simulink model "Final_test"  (R2018a)
settings: Solver=FixedStepAuto  StartTime=0.0  StopTime=inf  FixedStep=0.01  RelTol=1e-3  EnableMultiTasking=on
InitFcn:
  | set_param('Final_test/Output/Run Sim','Value','1');
  | set_param('Final_test/Motor Switch','Value','0');
  | set_param('Final_test/Automatic Control','Value','0');
  | %set_param('Final_test/Manual PWM','Gain','0');
undefined symbols (not defined in the file or in its folder): Discrete, sigbuilder_block, Time
libraries: simulink x3, arduinolib x3, ctrlSharedLib x1, dspstat3 x1
settings Model: SimulationMode=external  ExtModeTrigDuration=2  Creator=adiravishankara  LastModifiedBy=adiravishankara
settings SolverCC: AutoInsertRateTranBlk=on
settings OptimizationCC: EnhancedBackFolding=on  PassReuseOutputArgsThreshold=0  MaxStackSize=64  OptimizeBlockOrder=speed  DifferentSizesBufferReuse=on  OptimizationCustomize=off
settings DebuggingCC: ParameterTunabilityLossMsg=error
settings HardwareCC: ProdBitPerPointer=32  ProdBitPerSizeT=32  ProdBitPerPtrDiffT=32  ProdLargestAtomicInteger=Long  ProdLargestAtomicFloat=Double  ProdWordSize=32  ProdHWDeviceType=ARM Compatible->ARM Cortex  UseEmbeddedCoderFeatures=off
settings SFSimCC: MATLABDynamicMemAlloc=off
settings RTWCC: SystemTargetFile=ert.tlc  HardwareBoard=Arduino Due  TLCOptions=-aInlineSetEventsForThisBaseRateFcn=TLC_FALSE -aSuppressMultiTaskScheduler=TLC_FALSE -aRateBasedStepFcn=1  TemplateMakefile=ert_default_tmf  GenerateReport=on  Toolchain=Arduino ARM  BuildConfiguration=Faster Runs  LaunchReport=on
settings CodeAppCC: ForceParamTrailComments=on  OperatorAnnotations=on
settings ERTTargetCC: ERTCustomFileBanners=off  SupportContinuousTime=on  SupportNonInlinedSFcns=on  RemoveResetFunc=off  SupportVariableSizeSignals=on  ModelStepFunctionPrototypeControlCompliant=off  ExtMode=on  ExtModeMexArgs='127.0.0.1' 0 17725  ERTSrcFileBannerTemplate=codertarget_code_template.cgt  ERTHdrFileBannerTemplate=codertarget_code_template.cgt  ERTDataSrcFileTemplate=codertarget_code_template.cgt  ERTDataHdrFileTemplate=codertarget_code_template.cgt

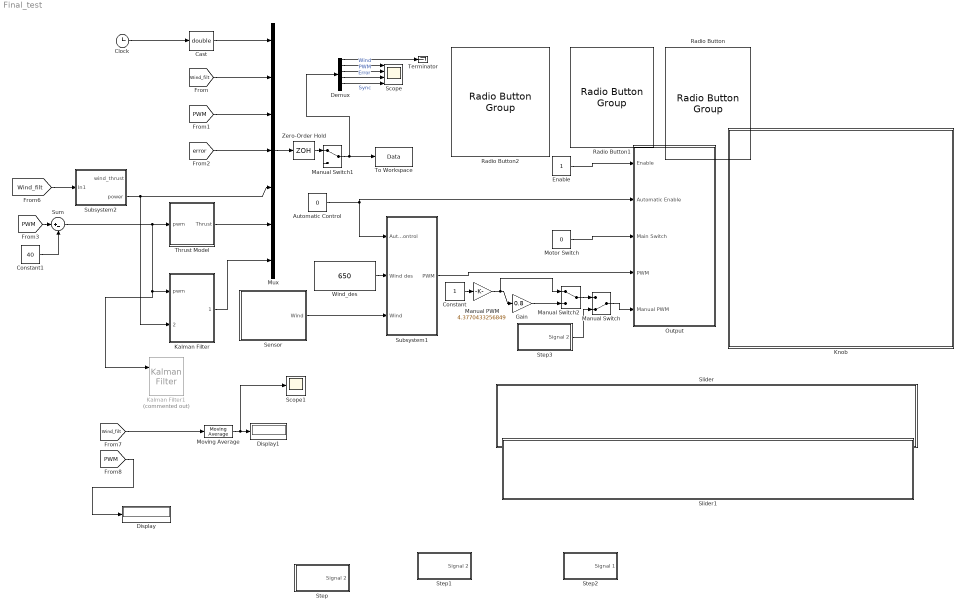
== system Final_test ==
  Automatic Control : Constant  Value=0  SampleTime=0.01
  Cast : DataTypeConversion  OutDataTypeStr=double
  Clock : Clock
  Constant : Constant  SampleTime=0.01
  Constant1 : Constant  Value=40
  Demux : Demux  Outputs=6
  Display : Display
  Display1 : Display
  Enable : Constant  SampleTime=0.01
  Gain : Gain  Gain=0.8
  Kalman Filter : Subsystem
  Kalman Filter1 : ctrlSharedLib/Kalman Filter  Commented=on  TimeDomain=Discrete-Time  UseCurrentEstimator=on  ModelSource=Individual A, B, C, D matrices  ModelSourceVariable=ss(0.95,1,1,0,1)  A="[0.9998  0.009851; -0.0394    0.9702]"  B=[0.000198; 0.0394]  C=[1 0]  D=0  NumberOfStates=1  NumberOfInputs=1  NumberOfOutputs=1  InitialEstimateSource=Dialog  X0=0  P0=10  UseK=off  UseGH=off  NumberOfProcessNoiseInputs=1  G=1  TimeInvariantG=on  H=0  TimeInvariantH=on  Q=1  TimeInvariantQ=on  R=5  TimeInvariantR=on  N=0  TimeInvariantN=on  AddInputPort=on  AddEnablePort=off  OutputEstimatedY=off  OutputP=off  Ts=-1
      settings: SourceProductBaseCode=CT
  Knob : Subsystem  DialogController=hmiCreateDDGDialog  IsWebBlock=on  mask(MWDashboardBlock){webBlockId=852d3d9e-f600-4180-8955-96c4171a0510, webBlockType=continuousknob, ShowInLibBrowser=on, ShowInitialText=on, HMISrcModelName=Final_test}
      mask prompts: webBlockId "WebBlock Id"; webBlockType "WebBlock Type"; HMISrcModelName "Source Model"
      mask help: SimulinkHMI:dialogs:ContinuousKnobDialogDesc
      mask Help: helpview([docroot '/mapfiles/simulink.map'], 'hmi_knob')
      mask Display:
      | if strcmp(get_param(bdroot(gcb),'BlockDiagramType'), 'library')
      |     image([(matlabroot) '/toolbox/simulink/hmi/icons/ContinuousKnob.png']);
      | end
  Manual PWM : Gain  Gain=4.3770433256849
  Manual Switch : ManualSwitch  CurrentSetting=0
  Manual Switch1 : ManualSwitch
  Manual Switch2 : ManualSwitch
  Motor Switch : Constant  Value=0  SampleTime=0.01
  Moving Average : dspstat3/Moving Average  Method=Sliding window  ForgettingFactorPort=off  SpecifyWindowLength=on  WindowLength=5  ForgettingFactor=0.9  SimulateUsing=Code generation
  Mux : Mux  Inputs=7
  Output : Subsystem
  Radio Button : RadioButtonGroup  WebBlockId=124  SelectedLabel=OFF  ButtonGroupName=SIM STATUS
      settings: Values={{'ON', 'OFF'}, [1 0]}
  Radio Button1 : RadioButtonGroup  WebBlockId=141  SelectedLabel=OFF  ButtonGroupName=SIM STATUS
      settings: Values={{'ON', 'OFF'}, [1 0]}
  Radio Button2 : RadioButtonGroup  WebBlockId=144  SelectedLabel=OFF  ButtonGroupName=SIM STATUS
      settings: Values={{'ON', 'OFF'}, [1 0]}
  Scope : Scope  NumInputPorts=4
  Scope1 : Scope
  Sensor : Subsystem
  Slider : Subsystem  DialogController=hmiCreateDDGDialog  IsWebBlock=on  mask(MWDashboardBlock){webBlockId=6d6bce73-9061-4720-a103-f9820fa904f8, webBlockType=slider, ShowInLibBrowser=on, ShowInitialText=on, HMISrcModelName=Final_test}
      mask prompts: webBlockId "WebBlock Id"; webBlockType "WebBlock Type"; HMISrcModelName "Source Model"
      mask help: SimulinkHMI:dialogs:SliderDialogDesc
      mask Help: helpview([docroot '/mapfiles/simulink.map'], 'hmi_slider')
      mask Display:
      | if strcmp(get_param(bdroot(gcb),'BlockDiagramType'), 'library')
      |     image([(matlabroot) '/toolbox/simulink/hmi/icons/Slider.png']);
      | end
  Slider1 : Subsystem  DialogController=hmiCreateDDGDialog  IsWebBlock=on  mask(MWDashboardBlock){webBlockId=583235cf-a666-476d-a93b-c374fcd1b609, webBlockType=slider, ShowInLibBrowser=on, ShowInitialText=on, HMISrcModelName=Final_test}
      mask prompts: webBlockId "WebBlock Id"; webBlockType "WebBlock Type"; HMISrcModelName "Source Model"
      mask help: SimulinkHMI:dialogs:SliderDialogDesc
      mask Help: helpview([docroot '/mapfiles/simulink.map'], 'hmi_slider')
      mask Display:
      | if strcmp(get_param(bdroot(gcb),'BlockDiagramType'), 'library')
      |     image([(matlabroot) '/toolbox/simulink/hmi/icons/Slider.png']);
      | end
  Step : Subsystem  Tag=STV Subsys  LoadFcn=sigbuilder_block('load');  StartFcn=sigbuilder_block('start');  StopFcn=sigbuilder_block('stop');  ClipboardFcn=sigbuilder_block('clipboard');  mask(Sigbuilder block){tuvar=[0:10]}
      mask help: Simulink:masks:SigbuilderBlock_MD
      mask init:
      | if ~strcmp(get_param(bdroot(gcbh),'SimulationStatus'),'stopped') tuvar = sigbuilder_block('maskInit'); end
      settings: CopyFcn=sigbuilder_block('copy');  DeleteFcn=sigbuilder_block('delete');  ModelCloseFcn=sigbuilder_block('modelClose');  PreSaveFcn=sigbuilder_block('preSave');  PauseFcn=sigbuilder_block('pause');  ContinueFcn=sigbuilder_block('continue');  NameChangeFcn=sigbuilder_block('namechange');  OpenFcn=sigbuilder_block('open',[48.75 0 1391.25 750.75 ]);  CloseFcn=sigbuilder_block('close');
      mask Display: plot(0, 0, 100, 100,[2, 2, 32, 32, 2], [68, 8, 8, 68, 68],[32, 2], [38, 38], [32, 19, 2],[53, 60, 44], [32, 17, 17, 2],[16, 16, 31, 31]);txt = getActiveGroup(gcbh);text(2, 100, txt,'verticalAlignment', 'top');
  Step1 : Subsystem  Tag=STV Subsys  LoadFcn=sigbuilder_block('load');  StartFcn=sigbuilder_block('start');  StopFcn=sigbuilder_block('stop');  ClipboardFcn=sigbuilder_block('clipboard');  mask(Sigbuilder block){tuvar=[0:10]}
      mask help: Simulink:masks:SigbuilderBlock_MD
      mask init:
      | if ~strcmp(get_param(bdroot(gcbh),'SimulationStatus'),'stopped') tuvar = sigbuilder_block('maskInit'); end
      settings: CopyFcn=sigbuilder_block('copy');  DeleteFcn=sigbuilder_block('delete');  ModelCloseFcn=sigbuilder_block('modelClose');  PreSaveFcn=sigbuilder_block('preSave');  PauseFcn=sigbuilder_block('pause');  ContinueFcn=sigbuilder_block('continue');  NameChangeFcn=sigbuilder_block('namechange');  OpenFcn=sigbuilder_block('open',[48.75 0 1391.25 729.75 ]);  CloseFcn=sigbuilder_block('close');
      mask Display: plot(0, 0, 100, 100,[2, 2, 32, 32, 2], [68, 8, 8, 68, 68],[32, 2], [38, 38], [32, 19, 2],[53, 60, 44], [32, 17, 17, 2],[16, 16, 31, 31]);txt = getActiveGroup(gcbh);text(2, 100, txt,'verticalAlignment', 'top');
  Step2 : Subsystem  Tag=STV Subsys  LoadFcn=sigbuilder_block('load');  StartFcn=sigbuilder_block('start');  StopFcn=sigbuilder_block('stop');  ClipboardFcn=sigbuilder_block('clipboard');  mask(Sigbuilder block){tuvar=[0:10]}
      mask help: Simulink:masks:SigbuilderBlock_MD
      mask init:
      | if ~strcmp(get_param(bdroot(gcbh),'SimulationStatus'),'stopped') tuvar = sigbuilder_block('maskInit'); end
      settings: CopyFcn=sigbuilder_block('copy');  DeleteFcn=sigbuilder_block('delete');  ModelCloseFcn=sigbuilder_block('modelClose');  PreSaveFcn=sigbuilder_block('preSave');  PauseFcn=sigbuilder_block('pause');  ContinueFcn=sigbuilder_block('continue');  NameChangeFcn=sigbuilder_block('namechange');  OpenFcn=sigbuilder_block('open',[48.75 1.5 1383.75 707.25 ]);  CloseFcn=sigbuilder_block('close');
      mask Display: plot(0, 0, 100, 100,[2, 2, 32, 32, 2], [68, 8, 8, 68, 68],[32, 2], [38, 38], [32, 19, 2],[53, 60, 44], [32, 17, 17, 2],[16, 16, 31, 31]);txt = getActiveGroup(gcbh);text(2, 100, txt,'verticalAlignment', 'top');
  Step3 : Subsystem  Tag=STV Subsys  LoadFcn=sigbuilder_block('load');  StartFcn=sigbuilder_block('start');  StopFcn=sigbuilder_block('stop');  ClipboardFcn=sigbuilder_block('clipboard');  mask(Sigbuilder block){tuvar=[0:10]}
      mask help: Simulink:masks:SigbuilderBlock_MD
      mask init:
      | if ~strcmp(get_param(bdroot(gcbh),'SimulationStatus'),'stopped') tuvar = sigbuilder_block('maskInit'); end
      settings: CopyFcn=sigbuilder_block('copy');  DeleteFcn=sigbuilder_block('delete');  ModelCloseFcn=sigbuilder_block('modelClose');  PreSaveFcn=sigbuilder_block('preSave');  PauseFcn=sigbuilder_block('pause');  ContinueFcn=sigbuilder_block('continue');  NameChangeFcn=sigbuilder_block('namechange');  OpenFcn=sigbuilder_block('open',[48.75 0 1391.25 729.75 ]);  CloseFcn=sigbuilder_block('close');
      mask Display: plot(0, 0, 100, 100,[2, 2, 32, 32, 2], [68, 8, 8, 68, 68],[32, 2], [38, 38], [32, 19, 2],[53, 60, 44], [32, 17, 17, 2],[16, 16, 31, 31]);txt = getActiveGroup(gcbh);text(2, 100, txt,'verticalAlignment', 'top');
  Subsystem1 : Subsystem
  Subsystem2 : Subsystem
  Sum : Sum  Inputs=|+-
  Terminator : Terminator
  Thrust Model : Subsystem
  To Workspace : ToWorkspace  VariableName=Data  SampleTime=-1
      settings: Save2DSignal=2-D array (concatenate along first dimension)
  Wind_des : Constant  Value=650  SampleTime=0.01
  Zero-Order Hold : ZeroOrderHold  SampleTime=0.01
  wires:
  Motor Switch/1 -> Output/3(Main Switch)
  Enable/1 -> Output/1(Enable)
  Constant/1 -> Manual PWM/1
  Wind_des/1 -> Subsystem1/2(Wind des)
  Subsystem1/1(PWM) -> Output/4(PWM)
  Automatic Control/1 -> Subsystem1/1(Automatic Control), Output/2(Automatic Enable)
  Sensor/1(Wind) -> Subsystem1/3(Wind)
  Mux/1 -> Zero-Order Hold/1
  [Wind_filt] -> Mux/2
  [PWM] -> Mux/3
  [error] -> Mux/4
  Clock/1 -> Cast/1
  Cast/1 -> Mux/1
  Manual Switch/1 -> Output/5(Manual PWM)
  Manual Switch1/1 -> Demux/1, To Workspace/1
  Zero-Order Hold/1 -> Manual Switch1/1
  Demux/2 -> Scope/1  "Wind"
  Demux/5 -> Scope/4  "Sync"
  Demux/4 -> Scope/3  "Error"
  Demux/3 -> Scope/2  "PWM"
  Demux/1 -> Terminator/1
  Constant1/1 -> Sum/2
  Sum/1 -> Kalman Filter1/1, Kalman Filter/1(pwm), Thrust Model/1(pwm)
  [Wind_filt] -> Subsystem2/1(In1)
  Thrust Model/1(Thrust) -> Mux/6
  [PWM] -> Sum/1
  Moving Average/1 -> Scope1/1, Display1/1
  [Wind_filt] -> Moving Average/1
  [PWM] -> Display/1
  Kalman Filter/1(Wind estimate) -> Mux/7
  Manual PWM/1 -> Gain/1, Manual Switch2/1
  Gain/1 -> Manual Switch2/2
  Manual Switch2/1 -> Manual Switch/1
  Subsystem2/2("power ") -> Kalman Filter/2(Wind_thrust), Mux/5
  Step3/1(Signal 2) -> Manual Switch/2

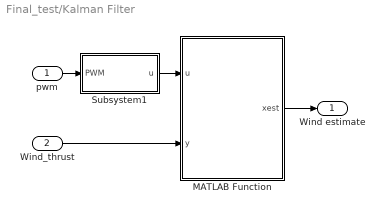
== system Final_test/Kalman Filter ==
  pwm : Inport
  Wind_thrust : Inport  Port=2
  MATLAB Function : MATLAB Function  TreatAsAtomicUnit=on
  Subsystem1 : Subsystem
  Wind estimate : Outport
  wires:
  Subsystem1/1(u) -> MATLAB Function/1(u)
  Wind_thrust/1 -> MATLAB Function/2(y)
  pwm/1 -> Subsystem1/1(PWM)
  MATLAB Function/1(xest) -> Wind estimate/1

== system Final_test/Knob ==

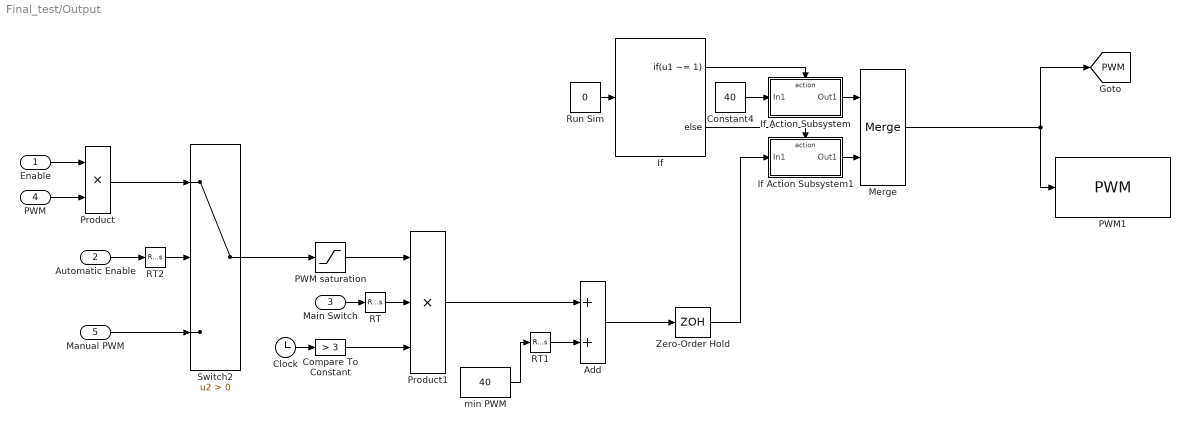
== system Final_test/Output ==
  Enable : Inport
  Automatic Enable : Inport  Port=2
  Main Switch : Inport  Port=3
  PWM : Inport  Port=4
  Manual PWM : Inport  Port=5
  Add : Sum
  Clock : Clock
      settings: Decimation=2
  Compare To Constant : simulink/Logic and Bit Operations/Compare To Constant  relop=>  const=3  OutDataTypeStr=boolean
  Constant4 : Constant  Value=40  SampleTime=0.01
  If : If  IfExpression=u1 ~= 1
  If Action Subsystem : Subsystem  TreatAsAtomicUnit=on
  If Action Subsystem1 : Subsystem  TreatAsAtomicUnit=on
  Merge : Merge
  PWM saturation : Saturate  UpperLimit=40  LowerLimit=0
  PWM1 : arduinolib/PWM  pinNumber=12  EnableInputFrequency=off  InitialFrequency=2000  InitialDutyCycle=0  NotificationType=None  blockPlatform=arduino
  Product : Product
  Product1 : Product  Inputs=3
  RT : RateTransition  OutPortSampleTime=0.01
  RT1 : RateTransition  OutPortSampleTime=0.01
  RT2 : RateTransition  OutPortSampleTime=0.01
  Run Sim : Constant  Value=0  SampleTime=0.01
  Switch2 : Switch  Criteria=u2 > Threshold
  Zero-Order Hold : ZeroOrderHold  SampleTime=0.01
  min PWM : Constant  Value=40  SampleTime=0.01
  tag scope: PWM=global
  wires:
  Clock/1 -> Compare To Constant/1
  min PWM/1 -> RT1/1
  Compare To Constant/1 -> Product1/3
  Automatic Enable/1 -> RT2/1
  Manual PWM/1 -> Switch2/3
  PWM/1 -> Product/2
  Switch2/1 -> PWM saturation/1
  Main Switch/1 -> RT/1
  Product1/1 -> Add/1
  PWM saturation/1 -> Product1/1
  Product/1 -> Switch2/1
  Enable/1 -> Product/1
  If/1 -> If Action Subsystem/Action
  Run Sim/1 -> If/1
  Constant4/1 -> If Action Subsystem/1(In1)
  Add/1 -> Zero-Order Hold/1
  If/2 -> If Action Subsystem1/Action
  If Action Subsystem1/1(Out1) -> Merge/2
  Merge/1 -> [PWM], PWM1/1
  Zero-Order Hold/1 -> If Action Subsystem1/1(In1)
  RT/1 -> Product1/2
  RT1/1 -> Add/2
  RT2/1 -> Switch2/2
  If Action Subsystem/1(Out1) -> Merge/1

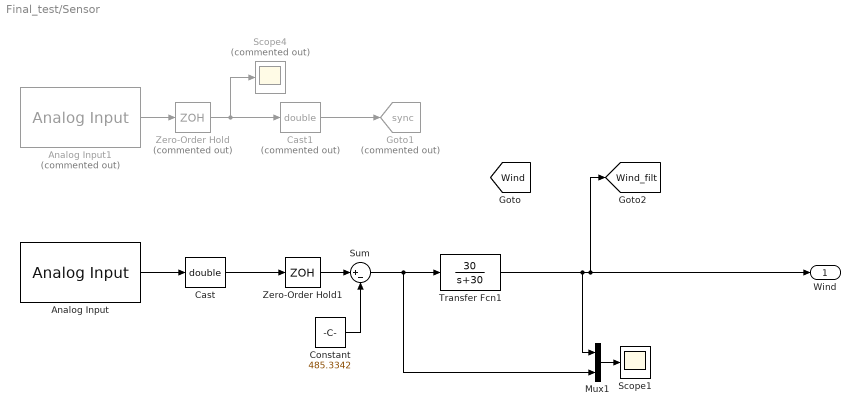
== system Final_test/Sensor ==
  Analog Input : arduinolib/Analog Input  pinNumber=2  ReadResultsOnly=off  ConversionTriggerSource=Software  ExternalTriggerType=uint32(0)  OutputDataType=uint16  EnableConversionCompleteNotify=off  EnableOuputStatus=off  SampleTime=0.01  blockPlatform=arduino
  Analog Input1 : arduinolib/Analog Input  Commented=on  pinNumber=3  ReadResultsOnly=off  ConversionTriggerSource=Software  ExternalTriggerType=uint32(0)  OutputDataType=uint16  EnableConversionCompleteNotify=off  EnableOuputStatus=off  SampleTime=0.01  blockPlatform=arduino
  Cast : DataTypeConversion  OutDataTypeStr=double
  Cast1 : DataTypeConversion  Commented=on  OutDataTypeStr=double
  Constant : Constant  Value=485.3342
  Goto1 : Goto  Commented=on  GotoTag=sync  TagVisibility=global
  Mux1 : Mux  Inputs=2
  Scope1 : Scope
  Scope4 : Scope  Commented=on
  Sum : Sum  Inputs=|+-
  Transfer Fcn1 : TransferFcn  Numerator=[30]  Denominator=[1 30]
  Zero-Order Hold : ZeroOrderHold  Commented=on  SampleTime=0.01
  Zero-Order Hold1 : ZeroOrderHold  SampleTime=0.01
  Wind : Outport
  tag scope: Wind=global, Wind_filt=global
  wires:
  Zero-Order Hold/1 -> Cast1/1, Scope4/1
  Analog Input/1 -> Cast/1
  Cast/1 -> Zero-Order Hold1/1
  Analog Input1/1 -> Zero-Order Hold/1
  Cast1/1 -> Goto1/1
  Zero-Order Hold1/1 -> Sum/1
  Transfer Fcn1/1 -> Mux1/1, [Wind_filt], Wind/1
  Mux1/1 -> Scope1/1
  Constant/1 -> Sum/2
  Sum/1 -> Mux1/2, Transfer Fcn1/1

== system Final_test/Slider ==

== system Final_test/Slider1 ==

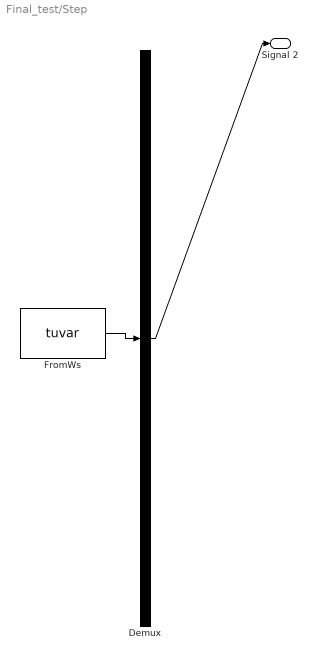
== system Final_test/Step ==
  Demux : Demux  Tag=STV Demux  Outputs=1
  FromWs : FromWorkspace  Tag=STV FromWs  VariableName=tuvar  SampleTime=0
      SigBuilderData=|
      | common.afterFinalStr = 'Extrapolate'
      | common.sampleTime = 0
      | dataSet.timeRange = [0 1700]
      | dataSet.name = 'Group 1'
      | sbobj.Groups.Name = 'Group 1'
      | sbobj.Groups.Signals.Name = 'Signal 2'
      | sbobj.Groups.Signals.XData = [0 29 29 59 89 119 149 179 209 209 239 269 299 389 389 570 570 750 750 930 930 1110 1110 1290 1290 1470 1470 1650 1650 1700]
      | sbobj.Groups.Signals.YData = [0 0 4 4 4 4 4 4 4 6 6 6 6 6 8 8 10 10 12 12 14 14 16 16 18 18 20 20 0 0]
      | sbobj.Groups.TimeRange = [0 1700]
  Signal 2 : Outport  Tag=STV Outport
  wires:
  FromWs/1 -> Demux/1
  Demux/1 -> Signal 2/1

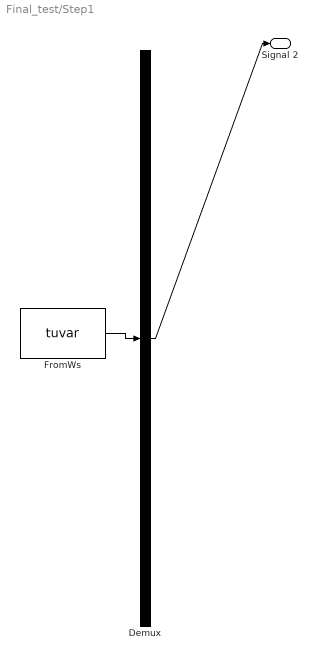
== system Final_test/Step1 ==
  Demux : Demux  Tag=STV Demux  Outputs=1
  FromWs : FromWorkspace  Tag=STV FromWs  VariableName=tuvar  SampleTime=0
      SigBuilderData=|
      | common.afterFinalStr = 'Extrapolate'
      | common.sampleTime = 0
      | dataSet.timeRange = [0 340]
      | dataSet.name = 'Group 1'
      | sbobj.Groups.Name = 'Group 1'
      | sbobj.Groups.Signals.Name = 'Signal 2'
      | sbobj.Groups.Signals.XData = [0 15 15 30 30 45 45 60 60 75 75 90 90 105 105 120 120 135 135 150 150 165 165 180 180 195 195 210 210 225 225 240 240 255 255 270 270 285 300 340]
      | sbobj.Groups.Signals.YData = [0 0 4 4 6 6 8 8 10 10 12 12 14 14 16 16 18 18 20 20 22 22 24 24 26 26 28 28 30 30 32 32 34 34 36 36 0 0 0 0]
      | sbobj.Groups.TimeRange = [0 340]
  Signal 2 : Outport  Tag=STV Outport
  wires:
  Demux/1 -> Signal 2/1
  FromWs/1 -> Demux/1

== system Final_test/Step2 ==
  Demux : Demux  Tag=STV Demux  Outputs=1
  FromWs : FromWorkspace  Tag=STV FromWs  VariableName=tuvar  SampleTime=0
      SigBuilderData=|
      | common.afterFinalStr = 'Extrapolate'
      | common.sampleTime = 0
      | dataSet.timeRange = [0 600]
      | dataSet.name = 'Group 1'
      | sbobj.Groups.Name = 'Group 1'
      | sbobj.Groups.Signals.Name = 'Signal 1'
      | sbobj.Groups.Signals.XData = [0 30 30 90 90 150 150 210 210 270 270 330 330 390 390 450 450 510 510 570 570 600]
      | sbobj.Groups.Signals.YData = [0 0 4 4 6 6 8 8 10 10 12 12 14 14 16 16 18 18 20 20 1 1]
      | sbobj.Groups.TimeRange = [0 600]
  Signal 1 : Outport  Tag=STV Outport
  wires:
  FromWs/1 -> Demux/1
  Demux/1 -> Signal 1/1

== system Final_test/Step3 ==
  Demux : Demux  Tag=STV Demux  Outputs=1
  FromWs : FromWorkspace  Tag=STV FromWs  VariableName=tuvar  SampleTime=0
      SigBuilderData=|
      | common.afterFinalStr = 'Extrapolate'
      | common.sampleTime = 0
      | dataSet.timeRange = [0 180]
      | dataSet.name = 'Group 1'
      | sbobj.Groups.Name = 'Group 1'
      | sbobj.Groups.Signals.Name = 'Signal 2'
      | sbobj.Groups.Signals.XData = [0 4 4 6 6 15 15 30 30 45 45 60 60 75 75 90 90 105 105 120 120 135 135 150 150 165 180]
      | sbobj.Groups.Signals.YData = [0 0 20 20 0 0 4 4 6 6 8 8 10 10 12 12 14 14 16 16 18 18 20 20 0 0 0]
      | sbobj.Groups.TimeRange = [0 180]
  Signal 2 : Outport  Tag=STV Outport
  wires:
  FromWs/1 -> Demux/1
  Demux/1 -> Signal 2/1

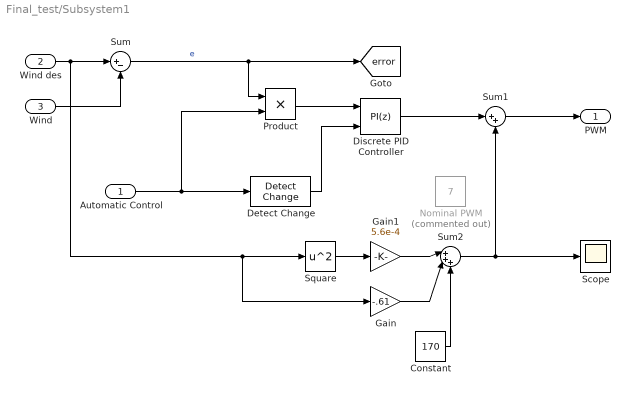
== system Final_test/Subsystem1 ==
  Automatic Control : Inport
  Wind des : Inport  Port=2
  Wind : Inport  Port=3
  Constant : Constant  Value=170
  Detect Change : simulink/Logic and Bit Operations/Detect Change  vinit=0  OutDataTypeStr=boolean
  Discrete PID Controller : simulink/Continuous/PID Controller  Controller=PI  TimeDomain=Discrete-time  SampleTime=0.01  IntegratorMethod=Forward Euler  FilterMethod=Forward Euler  Form=Parallel  UseFilter=on  ControllerParametersSource=internal  P=0.05  I=0.01  D=0  N=100  InitialConditionSource=internal  InitialConditionForIntegrator=0  InitialConditionForFilter=0  ExternalReset=rising  LimitOutput=off  UpperSaturationLimit=inf  LowerSaturationLimit=-inf  LinearizeAsGain=off  AntiWindupMode=none  Kb=1  TrackingMode=off  Kt=1  PParamMin=[]  PParamMax=[]  IParamMin=[]  IParamMax=[]  DParamMin=[]  DParamMax=[]  NParamMin=[]  NParamMax=[]  KbParamMin=[]  KbParamMax=[]  KtParamMin=[]  KtParamMax=[]  POutMin=[]  POutMax=[]  IOutMin=[]  IOutMax=[]  DOutMin=[]  DOutMax=[]  NOutMin=[]  NOutMax=[]  KbOutMin=[]  KbOutMax=[]  KtOutMin=[]  KtOutMax=[]  IntegratorOutMin=[]  IntegratorOutMax=[]  FilterOutMin=[]  FilterOutMax=[]  SumOutMin=[]  SumOutMax=[]  SumI1OutMin=[]  SumI1OutMax=[]  SumI2OutMin=[]  SumI2OutMax=[]  SumI3OutMin=[]  SumI3OutMax=[]  SumDOutMin=[]  SumDOutMax=[]  SaturationOutMin=[]  SaturationOutMax=[]  IntegratorContinuousStateAttributes=''  IntegratorStateMustResolveToSignalObject=off  IntegratorRTWStateStorageClass=Auto  FilterContinuousStateAttributes=''  FilterStateMustResolveToSignalObject=off  FilterRTWStateStorageClass=Auto  DifferentiatorICPrevScaledInput=0  DifferentiatorOutMin=[]  DifferentiatorOutMax=[]  FilterDiffOutCoefMin=[]  FilterDiffOutCoefMax=[]  SumDenOutMin=[]  SumDenOutMax=[]  SumNumOutMin=[]  SumNumOutMax=[]  ReciprocalOutMin=[]  ReciprocalOutMax=[]  DivideOutMin=[]  DivideOutMax=[]  TunerSelectOption=Transfer Function Based (PID Tuner App)
  Gain : Gain  Gain=-.61
  Gain1 : Gain  Gain=5.6e-4
  Nominal PWM : Constant  Commented=on  Value=7  SampleTime=0.01
  Product : Product
  Scope : Scope
  Square : Math  Operator=square  SaturateOnIntegerOverflow=on
  Sum : Sum  Inputs=|+-
  Sum1 : Sum  Inputs=|++
  Sum2 : Sum  Inputs=|+++
  PWM : Outport
  tag scope: error=global
  wires:
  Detect Change/1 -> Discrete PID Controller/2
  Wind des/1 -> Gain/1, Square/1, Sum/1
  Discrete PID Controller/1 -> Sum1/1
  Sum/1 -> [error], Product/1  "e"
  Wind/1 -> Sum/2
  Automatic Control/1 -> Product/2, Detect Change/1
  Sum1/1 -> PWM/1
  Product/1 -> Discrete PID Controller/1
  Gain/1 -> Sum2/2
  Gain1/1 -> Sum2/1
  Constant/1 -> Sum2/3
  Square/1 -> Gain1/1
  Sum2/1 -> Sum1/2, Scope/1

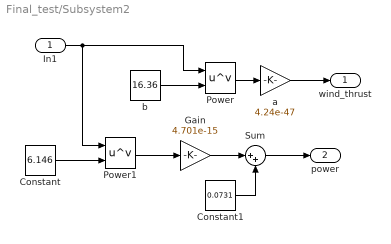
== system Final_test/Subsystem2 ==
  In1 : Inport
  Constant : Constant  Value=6.146
  Constant1 : Constant  Value=0.0731
  Gain : Gain  Gain=4.701e-15
  Power : Math  Operator=pow  SaturateOnIntegerOverflow=on
  Power1 : Math  Operator=pow  SaturateOnIntegerOverflow=on
  Sum : Sum  Inputs=|++
  a : Gain  Gain=4.24e-47
  b : Constant  Value=16.36
  "wind_thrust " : Outport
  "power " : Outport  Port=2
  wires:
  b/1 -> Power/2
  Power/1 -> a/1
  a/1 -> "wind_thrust "/1
  In1/1 -> Power1/1, Power/1
  Constant/1 -> Power1/2
  Power1/1 -> Gain/1
  Gain/1 -> Sum/1
  Constant1/1 -> Sum/2
  Sum/1 -> "power "/1

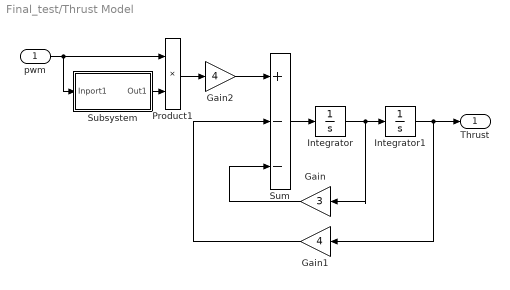
== system Final_test/Thrust Model ==
  pwm : Inport
  Gain : Gain  Gain=3
  Gain1 : Gain  Gain=4
  Gain2 : Gain  Gain=4
  Integrator : Integrator
  Integrator1 : Integrator
  Product1 : Product
  Subsystem : Subsystem
  Sum : Sum  Inputs=+--
  Thrust : Outport
  wires:
  Product1/1 -> Gain2/1
  pwm/1 -> Product1/1, Subsystem/1(Inport1)
  Integrator/1 -> Gain/1, Integrator1/1
  Subsystem/1(Out1) -> Product1/2
  Sum/1 -> Integrator/1
  Integrator1/1 -> Gain1/1, Thrust/1
  Gain/1 -> Sum/3
  Gain1/1 -> Sum/2
  Gain2/1 -> Sum/1

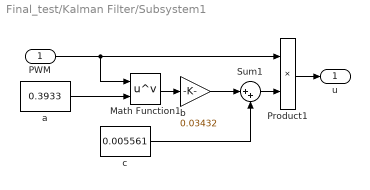
== system Final_test/Kalman Filter/Subsystem1 ==
  PWM : Inport
  Math Function1 : Math  Operator=pow  SaturateOnIntegerOverflow=on
  Product1 : Product
  Sum1 : Sum  Inputs=|++
  a : Constant  Value=0.3933
  b : Gain  Gain=0.03432
  c : Constant  Value=0.005561
  u : Outport
  wires:
  Sum1/1 -> Product1/2
  Product1/1 -> u/1
  a/1 -> Math Function1/2
  b/1 -> Sum1/1
  PWM/1 -> Math Function1/1, Product1/1
  Math Function1/1 -> b/1
  c/1 -> Sum1/2

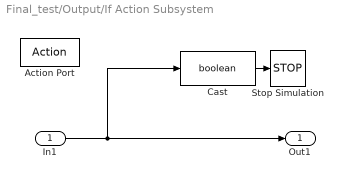
== system Final_test/Output/If Action Subsystem ==
  In1 : Inport
  Action Port : ActionPort  ActionType=then
  Cast : DataTypeConversion  OutDataTypeStr=boolean
  Stop Simulation : Stop
  Out1 : Outport
  wires:
  In1/1 -> Cast/1, Out1/1
  Cast/1 -> Stop Simulation/1

== system Final_test/Output/If Action Subsystem1 ==
  In1 : Inport
  Action Port : ActionPort  ActionType=else
  Out1 : Outport
  wires:
  In1/1 -> Out1/1

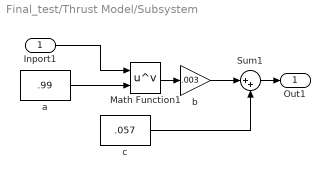
== system Final_test/Thrust Model/Subsystem ==
  Inport1 : Inport
  Math Function1 : Math  Operator=pow  SaturateOnIntegerOverflow=on
  Sum1 : Sum  Inputs=|++
  a : Constant  Value=.99
  b : Gain  Gain=.003
  c : Constant  Value=.057
  Out1 : Outport
  wires:
  a/1 -> Math Function1/2
  b/1 -> Sum1/1
  Inport1/1 -> Math Function1/1
  Math Function1/1 -> b/1
  Sum1/1 -> Out1/1
  c/1 -> Sum1/2

== matlab function Final_test/Kalman Filter/MATLAB Function ==
  settings: updateMethod=DISCRETE
  data: u input; xest output; y input
function xest  = fcn(u, y)
persistent P xh
if isempty(P)
    P = eye(2);
    xh = zeros(2,1);
end
% A = [0 1; -4 -3];
% B = [0; 4];
% C = [1 0];

Ad = [0.9998  0.009851; -0.0394    0.9702];
Bd = [0.000198; 0.0394];
Cd = [1 0];

Q = 1;
R = diag([5,5]);


% Model information
xh_bar = Ad * xh + Bd * u;
P_bar = Ad * P * Ad' + R;

% Measurement update
K = P_bar * Cd' * (Cd * P_bar * Cd' + Q)^-1;
xh = xh_bar + K * (y - Cd * xh_bar);
P = (1 - K * Cd) * P_bar;

xest = xh;
